simulink model "testbench_stateflow_18a"  (R2019a)
settings: Solver=FixedStepDiscrete  StartTime=0.0  StopTime=inf  FixedStep=0.01  RelTol=1e-3  EnableMultiTasking=on
libraries: simulink x5
settings Model: Creator=Schneider  LastModifiedBy=YUMU
settings DataIOCC: LimitDataPoints=on  ReturnWorkspaceOutputs=off
settings OptimizationCC: LifeSpan=inf
settings DebuggingCC: AllowSymbolicDim=off  SFUnexpectedBacktrackingDiag=warning  SFNoUnconditionalDefaultTransitionDiag=warning  SFExecutionAtInitializationDiag=none  ArithmeticOperatorsInVariantConditions=warning
settings ModelReferenceCC: PropagateSignalLabelsOutOfModel=off
settings SFSimCC: SimUseLocalCustomCode=off
settings RTWCC: RTWUseLocalCustomCode=off
settings CodeAppCC: StateflowObjectComments=on
settings GRTTargetCC: TargetLangStandard=C89/C90 (ANSI)
settings ConfigComp: CovMetricSettings=dw  CovHtmlReporting=on  CovSaveCumulativeToWorkspaceVar=on  CovSaveSingleToWorkspaceVar=on  CovExternalEMLEnable=off

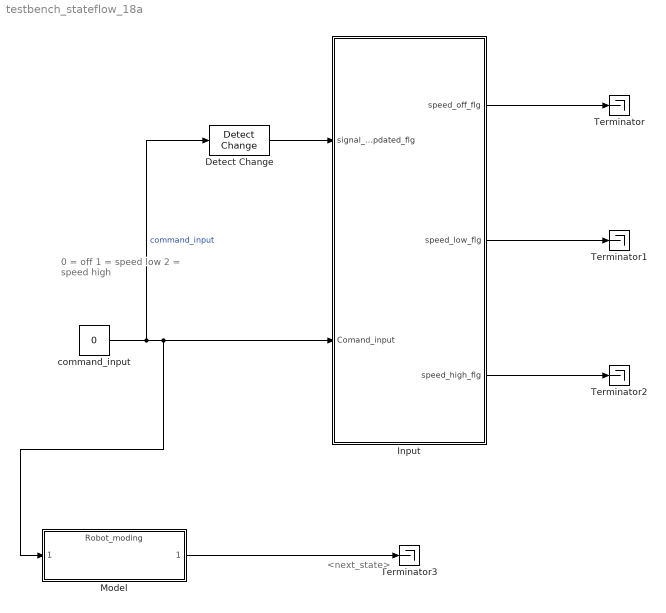
== system testbench_stateflow_18a ==
  note: <next_state>
  note: 0 = off
      | 1 = speed low
      | 2 = speed high
  Detect Change : simulink/Logic and Bit Operations/Detect Change  vinit=0  OutDataTypeStr=boolean
  Input : Subsystem
  Model : ModelReference  ModelNameDialog=Robot_moding  SimulationMode=Normal  ModelReferenceVersion=1.20
  Terminator{,1..3} (4 alike) : Terminator
  command_input : Constant  Value=0  OutDataTypeStr=uint8
  wires:
  Input/3(speed_high_flg) -> Terminator2/1
  Input/2(speed_low_flg) -> Terminator1/1
  Input/1(speed_off_flg) -> Terminator/1
  command_input/1 -> Detect Change/1, Model/1, Input/2(" Comand_input")  "command_input"
  Detect Change/1 -> Input/1(" signal_updated_flg")
  Model/1 -> Terminator3/1

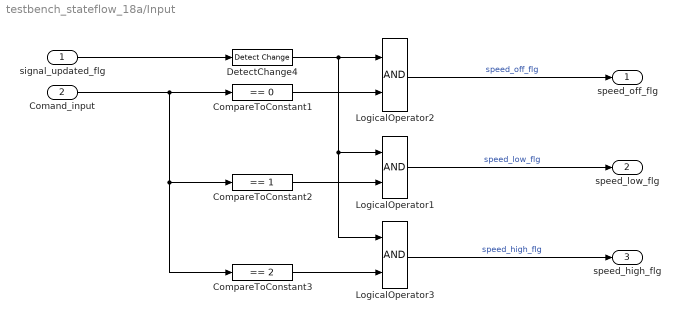
== system testbench_stateflow_18a/Input ==
  " signal_updated_flg" : Inport
  " Comand_input" : Inport  Port=2
  CompareToConstant1 : simulink/Logic and Bit Operations/Compare To Constant  relop===  const=0  OutDataTypeStr=boolean
  CompareToConstant2 : simulink/Logic and Bit Operations/Compare To Constant  relop===  const=1  OutDataTypeStr=boolean
  CompareToConstant3 : simulink/Logic and Bit Operations/Compare To Constant  relop===  const=2  OutDataTypeStr=boolean
  DetectChange4 : simulink/Logic and Bit Operations/Detect Change  vinit=0  OutDataTypeStr=boolean
  LogicalOperator1 : Logic  AllPortsSameDT=off  OutDataTypeStr=boolean
  LogicalOperator2 : Logic  AllPortsSameDT=off  OutDataTypeStr=boolean
  LogicalOperator3 : Logic  AllPortsSameDT=off  OutDataTypeStr=boolean
  speed_off_flg : Outport  OutDataTypeStr=boolean
  speed_low_flg : Outport  Port=2  OutDataTypeStr=boolean
  speed_high_flg : Outport  Port=3  OutDataTypeStr=boolean
  wires:
  LogicalOperator3/1 -> speed_high_flg/1  "speed_high_flg"
  LogicalOperator1/1 -> speed_low_flg/1  "speed_low_flg"
  LogicalOperator2/1 -> speed_off_flg/1  "speed_off_flg"
  " Comand_input"/1 -> CompareToConstant3/1, CompareToConstant2/1, CompareToConstant1/1
  CompareToConstant1/1 -> LogicalOperator2/2
  CompareToConstant3/1 -> LogicalOperator3/2
  CompareToConstant2/1 -> LogicalOperator1/2
  " signal_updated_flg"/1 -> DetectChange4/1
  DetectChange4/1 -> LogicalOperator3/1, LogicalOperator1/1, LogicalOperator2/1
